simulink subsystem "INV_PWMsyncTask"  (R2022b)
settings: Solver=VariableStepAuto  StartTime=0.0  StopTime=10.0  RelTol=1e-3
values from neighbouring files (symbols this model uses):
  DPWM0Duclamp = [0 0 0 0 0 0 0 0 0 0 0 0 ... (1024 elements, 1024x1)]    [PWMLookUp.mat]    (also in prep_DPWM0_table.m = uint8(DPWM0Duclamp))
  DPWM0Dufi = [12288 12331 12374 12417 12458 12500 12541 12581 12621 12661 12700 12739 ... (1024 elements, 1024x1)]    [PWMLookUp.mat]    (also in prep_DPWM0_table.m = storedInteger(fixedPointValue))
  DPWM0Dusecfi = [-8192 -8192 -8192 -8192 -8192 -8192 -8192 -8192 -8192 -8192 -8192 -8192 ... (1024 elements, 1024x1)]    [PWMLookUp.mat]    (also in prep_DPWM0_table.m = storedInteger(fixedPointValue))
  DPWM0Dvclamp = [0 0 0 0 0 0 0 0 0 0 0 0 ... (1024 elements, 1024x1)]    [PWMLookUp.mat]    (also in prep_DPWM0_table.m = uint8(DPWM0Dvclamp))
  DPWM0Dvfi = [0 87 174 261 348 435 522 609 696 783 870 957 ... (1024 elements, 1024x1)]    [PWMLookUp.mat]    (also in prep_DPWM0_table.m = storedInteger(fixedPointValue))
  DPWM0Dvsecfi = [-8192 -8192 -8192 -8192 -8192 -8192 -8192 -8192 -8192 -8192 -8192 -8192 ... (1024 elements, 1024x1)]    [PWMLookUp.mat]    (also in prep_DPWM0_table.m = storedInteger(fixedPointValue))
  DPWM0Dwclamp = [2 2 2 2 2 2 2 2 2 2 2 2 ... (1024 elements, 1024x1)]    [PWMLookUp.mat]    (also in prep_DPWM0_table.m = uint8(DPWM0Dwclamp))
  DPWM0Dwfi = [0 0 0 0 0 0 0 0 0 0 0 0 ... (1024 elements, 1024x1)]    [PWMLookUp.mat]    (also in prep_DPWM0_table.m = storedInteger(fixedPointValue))
  DPWM0Dwsecfi = [-8192 -8192 -8192 -8192 -8192 -8192 -8192 -8192 -8192 -8192 -8192 -8192 ... (1024 elements, 1024x1)]    [PWMLookUp.mat]    (also in prep_DPWM0_table.m = storedInteger(fixedPointValue))
  DPWM1Duclamp = [1 1 1 1 1 1 1 1 1 1 1 1 ... (1024 elements, 1024x1)]    [PWMLookUp.mat]    (also in prep_DPWM1_table.m = uint8(DPWM1Duclamp))
  DPWM1Dufi = [0 0 0 0 0 0 0 0 0 0 0 0 ... (1024 elements, 1024x1)]    [PWMLookUp.mat]    (also in prep_DPWM1_table.m = storedInteger(fixedPointValue))
  DPWM1Dusecfi = [8192 8192 8192 8192 8192 8192 8192 8192 8192 8192 8192 8192 ... (1024 elements, 1024x1)]    [PWMLookUp.mat]    (also in prep_DPWM1_table.m = storedInteger(fixedPointValue))
  DPWM1Dvclamp = [0 0 0 0 0 0 0 0 0 0 0 0 ... (1024 elements, 1024x1)]    [PWMLookUp.mat]    (also in prep_DPWM1_table.m = uint8(DPWM1Dvclamp))
  DPWM1Dvfi = [-12288 -12244 -12200 -12155 -12110 -12065 -12019 -11972 -11925 -11878 -11830 -11782 ... (1024 elements, 1024x1)]    [PWMLookUp.mat]    (also in prep_DPWM1_table.m = storedInteger(fixedPointValue))
  DPWM1Dvsecfi = [8192 8192 8192 8192 8192 8192 8192 8192 8192 8192 8192 8192 ... (1024 elements, 1024x1)]    [PWMLookUp.mat]    (also in prep_DPWM1_table.m = storedInteger(fixedPointValue))
  DPWM1Dwclamp = [0 0 0 0 0 0 0 0 0 0 0 0 ... (1024 elements, 1024x1)]    [PWMLookUp.mat]    (also in prep_DPWM1_table.m = uint8(DPWM1Dwclamp))
  DPWM1Dwfi = [-12288 -12331 -12374 -12417 -12458 -12500 -12541 -12581 -12621 -12661 -12700 -12739 ... (1024 elements, 1024x1)]    [PWMLookUp.mat]    (also in prep_DPWM1_table.m = storedInteger(fixedPointValue))
  DPWM1Dwsecfi = [8192 8192 8192 8192 8192 8192 8192 8192 8192 8192 8192 8192 ... (1024 elements, 1024x1)]    [PWMLookUp.mat]    (also in prep_DPWM1_table.m = storedInteger(fixedPointValue))
  DPWM2Duclamp = [1 1 1 1 1 1 1 1 1 1 1 1 ... (1024 elements, 1024x1)]    [PWMLookUp.mat]    (also in prep_DPWM2_table.m = uint8(DPWM2Duclamp))
  DPWM2Dufi = [0 0 0 0 0 0 0 0 0 0 0 0 ... (1024 elements, 1024x1)]    [PWMLookUp.mat]    (also in prep_DPWM2_table.m = storedInteger(fixedPointValue))
  DPWM2Dusecfi = [8192 8192 8192 8192 8192 8192 8192 8192 8192 8192 8192 8192 ... (1024 elements, 1024x1)]    [PWMLookUp.mat]    (also in prep_DPWM2_table.m = storedInteger(fixedPointValue))
  DPWM2Dvclamp = [0 0 0 0 0 0 0 0 0 0 0 0 ... (1024 elements, 1024x1)]    [PWMLookUp.mat]    (also in prep_DPWM2_table.m = uint8(DPWM2Dvclamp))
  DPWM2Dvfi = [-12288 -12244 -12200 -12155 -12110 -12065 -12019 -11972 -11925 -11878 -11830 -11782 ... (1024 elements, 1024x1)]    [PWMLookUp.mat]    (also in prep_DPWM2_table.m = storedInteger(fixedPointValue))
  DPWM2Dvsecfi = [8192 8192 8192 8192 8192 8192 8192 8192 8192 8192 8192 8192 ... (1024 elements, 1024x1)]    [PWMLookUp.mat]    (also in prep_DPWM2_table.m = storedInteger(fixedPointValue))
  DPWM2Dwclamp = [0 0 0 0 0 0 0 0 0 0 0 0 ... (1024 elements, 1024x1)]    [PWMLookUp.mat]    (also in prep_DPWM2_table.m = uint8(DPWM2Dwclamp))
  DPWM2Dwfi = [-12288 -12331 -12374 -12417 -12458 -12500 -12541 -12581 -12621 -12661 -12700 -12739 ... (1024 elements, 1024x1)]    [PWMLookUp.mat]    (also in prep_DPWM2_table.m = storedInteger(fixedPointValue))
  DPWM2Dwsecfi = [8192 8192 8192 8192 8192 8192 8192 8192 8192 8192 8192 8192 ... (1024 elements, 1024x1)]    [PWMLookUp.mat]    (also in prep_DPWM2_table.m = storedInteger(fixedPointValue))
  DPWM3Duclamp = [0 0 0 0 0 0 0 0 0 0 0 0 ... (1024 elements, 1024x1)]    [PWMLookUp.mat]    (also in prep_DPWM3_table.m = uint8(DPWM3Duclamp))
  DPWM3Dufi = [12288 12331 12374 12417 12458 12500 12541 12581 12621 12661 12700 12739 ... (1024 elements, 1024x1)]    [PWMLookUp.mat]    (also in prep_DPWM3_table.m = storedInteger(fixedPointValue))
  DPWM3Dusecfi = [-8192 -8192 -8192 -8192 -8192 -8192 -8192 -8192 -8192 -8192 -8192 -8192 ... (1024 elements, 1024x1)]    [PWMLookUp.mat]    (also in prep_DPWM3_table.m = storedInteger(fixedPointValue))
  DPWM3Dvclamp = [0 0 0 0 0 0 0 0 0 0 0 0 ... (1024 elements, 1024x1)]    [PWMLookUp.mat]    (also in prep_DPWM3_table.m = uint8(DPWM3Dvclamp))
  DPWM3Dvfi = [0 87 174 261 348 435 522 609 696 783 870 957 ... (1024 elements, 1024x1)]    [PWMLookUp.mat]    (also in prep_DPWM3_table.m = storedInteger(fixedPointValue))
  DPWM3Dvsecfi = [-8192 -8192 -8192 -8192 -8192 -8192 -8192 -8192 -8192 -8192 -8192 -8192 ... (1024 elements, 1024x1)]    [PWMLookUp.mat]    (also in prep_DPWM3_table.m = storedInteger(fixedPointValue))
  DPWM3Dwclamp = [2 2 2 2 2 2 2 2 2 2 2 2 ... (1024 elements, 1024x1)]    [PWMLookUp.mat]    (also in prep_DPWM3_table.m = uint8(DPWM3Dwclamp))
  DPWM3Dwfi = [0 0 0 0 0 0 0 0 0 0 0 0 ... (1024 elements, 1024x1)]    [PWMLookUp.mat]    (also in prep_DPWM3_table.m = storedInteger(fixedPointValue))
  DPWM3Dwsecfi = [-8192 -8192 -8192 -8192 -8192 -8192 -8192 -8192 -8192 -8192 -8192 -8192 ... (1024 elements, 1024x1)]    [PWMLookUp.mat]    (also in prep_DPWM3_table.m = storedInteger(fixedPointValue))
  DPWMmaxDuclamp = [1 1 1 1 1 1 1 1 1 1 1 1 ... (1024 elements, 1024x1)]    [PWMLookUp.mat]    (also in prep_DPWMmax_table.m = uint8(DPWMmaxDuclamp))
  DPWMmaxDufi = [0 0 0 0 0 0 0 0 0 0 0 0 ... (1024 elements, 1024x1)]    [PWMLookUp.mat]    (also in prep_DPWMmax_table.m = storedInteger(fixedPointValue))
  DPWMmaxDusecfi = [8192 8192 8192 8192 8192 8192 8192 8192 8192 8192 8192 8192 ... (1024 elements, 1024x1)]    [PWMLookUp.mat]    (also in prep_DPWMmax_table.m = storedInteger(fixedPointValue))
  DPWMmaxDvclamp = [0 0 0 0 0 0 0 0 0 0 0 0 ... (1024 elements, 1024x1)]    [PWMLookUp.mat]    (also in prep_DPWMmax_table.m = uint8(DPWMmaxDvclamp))
  DPWMmaxDvfi = [-12288 -12244 -12200 -12155 -12110 -12065 -12019 -11972 -11925 -11878 -11830 -11782 ... (1024 elements, 1024x1)]    [PWMLookUp.mat]    (also in prep_DPWMmax_table.m = storedInteger(fixedPointValue))
  DPWMmaxDvsecfi = [8192 8192 8192 8192 8192 8192 8192 8192 8192 8192 8192 8192 ... (1024 elements, 1024x1)]    [PWMLookUp.mat]    (also in prep_DPWMmax_table.m = storedInteger(fixedPointValue))
  DPWMmaxDwclamp = [0 0 0 0 0 0 0 0 0 0 0 0 ... (1024 elements, 1024x1)]    [PWMLookUp.mat]    (also in prep_DPWMmax_table.m = uint8(DPWMmaxDwclamp))
  DPWMmaxDwfi = [-12288 -12331 -12374 -12417 -12458 -12500 -12541 -12581 -12621 -12661 -12700 -12739 ... (1024 elements, 1024x1)]    [PWMLookUp.mat]    (also in prep_DPWMmax_table.m = storedInteger(fixedPointValue))
  DPWMmaxDwsecfi = [8192 8192 8192 8192 8192 8192 8192 8192 8192 8192 8192 8192 ... (1024 elements, 1024x1)]    [PWMLookUp.mat]    (also in prep_DPWMmax_table.m = storedInteger(fixedPointValue))
  DPWMminDuclamp = [0 0 0 0 0 0 0 0 0 0 0 0 ... (1024 elements, 1024x1)]    [PWMLookUp.mat]    (also in prep_DPWMmin_table.m = uint8(DPWMminDuclamp))
  DPWMminDufi = [12288 12331 12374 12417 12458 12500 12541 12581 12621 12661 12700 12739 ... (1024 elements, 1024x1)]    [PWMLookUp.mat]    (also in prep_DPWMmin_table.m = storedInteger(fixedPointValue))
  DPWMminDusecfi = [-8192 -8192 -8192 -8192 -8192 -8192 -8192 -8192 -8192 -8192 -8192 -8192 ... (1024 elements, 1024x1)]    [PWMLookUp.mat]    (also in prep_DPWMmin_table.m = storedInteger(fixedPointValue))
  DPWMminDvclamp = [0 0 0 0 0 0 0 0 0 0 0 0 ... (1024 elements, 1024x1)]    [PWMLookUp.mat]    (also in prep_DPWMmin_table.m = uint8(DPWMminDvclamp))
  DPWMminDvfi = [0 87 174 261 348 435 522 609 696 783 870 957 ... (1024 elements, 1024x1)]    [PWMLookUp.mat]    (also in prep_DPWMmin_table.m = storedInteger(fixedPointValue))
  DPWMminDvsecfi = [-8192 -8192 -8192 -8192 -8192 -8192 -8192 -8192 -8192 -8192 -8192 -8192 ... (1024 elements, 1024x1)]    [PWMLookUp.mat]    (also in prep_DPWMmin_table.m = storedInteger(fixedPointValue))
  DPWMminDwclamp = [2 2 2 2 2 2 2 2 2 2 2 2 ... (1024 elements, 1024x1)]    [PWMLookUp.mat]    (also in prep_DPWMmin_table.m = uint8(DPWMminDwclamp))
  DPWMminDwfi = [0 0 0 0 0 0 0 0 0 0 0 0 ... (1024 elements, 1024x1)]    [PWMLookUp.mat]    (also in prep_DPWMmin_table.m = storedInteger(fixedPointValue))
  DPWMminDwsecfi = [-8192 -8192 -8192 -8192 -8192 -8192 -8192 -8192 -8192 -8192 -8192 -8192 ... (1024 elements, 1024x1)]    [PWMLookUp.mat]    (also in prep_DPWMmin_table.m = storedInteger(fixedPointValue))
  SPWMDufi = [8192 8192 8191 8191 8190 8188 8186 8184 8182 8180 8177 8173 ... (1024 elements, 1024x1)]    [PWMLookUp.mat]    (also in prep_SinePWM_table.m = storedInteger(fixedPointValue))
  SPWMDvfi = [-4096 -4052 -4009 -3965 -3921 -3876 -3832 -3788 -3743 -3698 -3653 -3608 ... (1024 elements, 1024x1)]    [PWMLookUp.mat]    (also in prep_SinePWM_table.m = storedInteger(fixedPointValue))
  SPWMDwfi = [-4096 -4139 -4183 -4226 -4269 -4312 -4354 -4397 -4439 -4481 -4523 -4565 ... (1024 elements, 1024x1)]    [PWMLookUp.mat]    (also in prep_SinePWM_table.m = storedInteger(fixedPointValue))
  SVPWMDufi = [6144 6166 6187 6208 6229 6250 6270 6291 6311 6330 6350 6369 ... (1024 elements, 1024x1)]    [PWMLookUp.mat]    (also in prep_SVPWM_table.m = storedInteger(fixedPointValue))
  SVPWMDvfi = [-6144 -6079 -6013 -5947 -5881 -5815 -5748 -5681 -5614 -5547 -5480 -5412 ... (1024 elements, 1024x1)]    [PWMLookUp.mat]    (also in prep_SVPWM_table.m = storedInteger(fixedPointValue))
  SVPWMDwfi = [-6144 -6166 -6187 -6208 -6229 -6250 -6270 -6291 -6311 -6330 -6350 -6369 ... (1024 elements, 1024x1)]    [PWMLookUp.mat]    (also in prep_SVPWM_table.m = storedInteger(fixedPointValue))
  THISPWMDufi = [6823 6823 6823 6823 6824 6825 6826 6827 6828 6829 6831 6832 ... (1024 elements, 1024x1)]    [PWMLookUp.mat]    (also in prep_THISPWM_table.m = storedInteger(fixedPointValue))
  THISPWMDvfi = [-5465 -5421 -5377 -5332 -5286 -5240 -5193 -5145 -5097 -5049 -4999 -4949 ... (1024 elements, 1024x1)]    [PWMLookUp.mat]    (also in prep_THISPWM_table.m = storedInteger(fixedPointValue))
  THISPWMDwfi = [-5465 -5508 -5551 -5593 -5634 -5675 -5715 -5755 -5794 -5832 -5869 -5906 ... (1024 elements, 1024x1)]    [PWMLookUp.mat]    (also in prep_THISPWM_table.m = storedInteger(fixedPointValue))
libraries: simulink x16
(part 1 of 2)
settings Model: Creator=ReiterTo  LastModifiedBy=ReiterTo

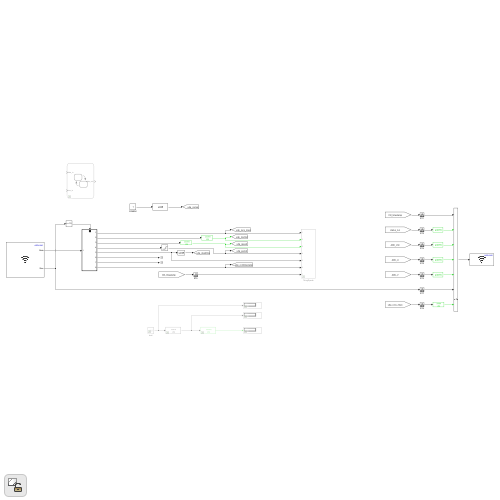
[thumbnail: Simulink's stored preview of the top-level diagram]
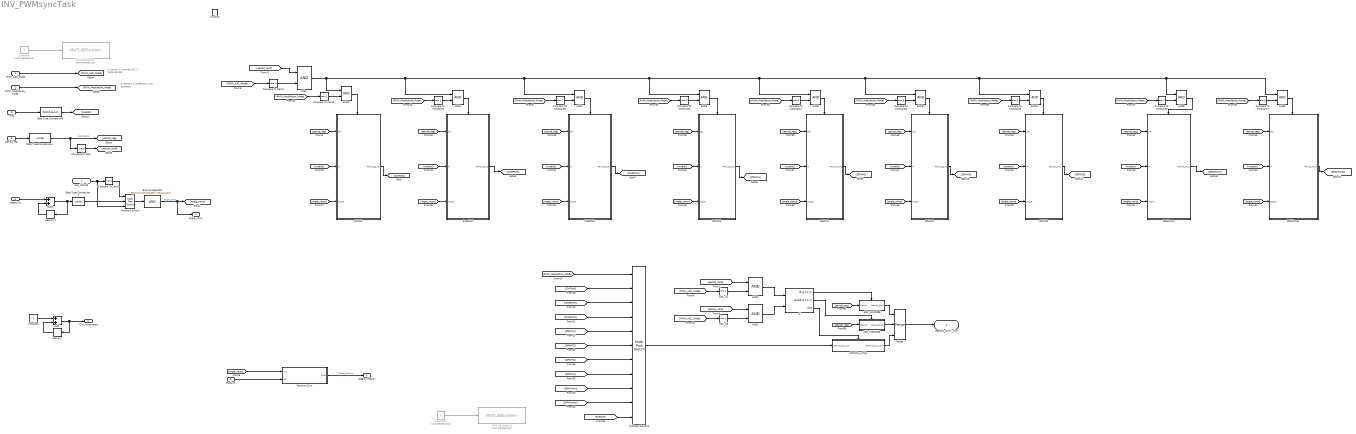
== system INV_PWMsyncTask ==
  note: 0: SVPWM
      | 1: SinePWM
      | 2: not available
  note: 0: normal
      | 1: lowside ASC
      | 2: highside ASC
  PWM_ASC_Mode : Inport  OutDataTypeStr=uint8  PortDimensions=1
  PWM_Modulation_Mode : Inport  Port=2  OutDataTypeStr=uint8  PortDimensions=1
  mod : Inport  Port=3  OutDataTypeStr=fixdt(0,16,14)  PortDimensions=1
  speed_inc : Inport  Port=4  OutDataTypeStr=fixdt(0,32,16)  PortDimensions=1
  period_reg : Inport  Port=5  OutDataTypeStr=uint16  PortDimensions=1
  PosSync : Inport  Port=6  OutDataTypeStr=uint16  PortDimensions=1
  pos_hillhold : Inport  Port=7  OutDataTypeStr=uint16  PortDimensions=1
  function : TriggerPort  TriggerType=function-call  VariantControl=(inherit)  PortDimensions=1
  AND{,1..11} (12 alike) : Logic  AllPortsSameDT=off  OutDataTypeStr=boolean
  ASC_HIGHSIDE : Subsystem  TreatAsAtomicUnit=on
  ASC_HS : simulink/Logic and Bit Operations/Compare To Constant  relop===  const=2  OutDataTypeStr=boolean
  ASC_LOWSIDE : Subsystem  TreatAsAtomicUnit=on
  ASC_LS : simulink/Logic and Bit Operations/Compare To Constant  relop===  const=1  OutDataTypeStr=boolean
  Add : Sum
  Add1 : Sum
  Bitwise Operator : simulink/Logic and Bit Operations/Bitwise Operator  logicop=AND  UseBitMask=on  BitMask=bin2dec('1111111111')  BitMaskRealWorld=Stored Integer
  Compare To Constant2 : simulink/Logic and Bit Operations/Compare To Constant  relop===  const=1  OutDataTypeStr=boolean
  Compare To Constant3 : simulink/Logic and Bit Operations/Compare To Constant  relop===  const=3  OutDataTypeStr=boolean
  Compare To Constant4 : simulink/Logic and Bit Operations/Compare To Constant  relop===  const=4  OutDataTypeStr=boolean
  Compare To Constant5 : simulink/Logic and Bit Operations/Compare To Constant  relop===  const=2  OutDataTypeStr=boolean
  Compare To Constant6 : simulink/Logic and Bit Operations/Compare To Constant  relop===  const=7  OutDataTypeStr=boolean
  Compare To Constant7 : simulink/Logic and Bit Operations/Compare To Constant  relop===  const=8  OutDataTypeStr=boolean
  Compare To Constant8 : simulink/Logic and Bit Operations/Compare To Constant  relop===  const=5  OutDataTypeStr=boolean
  Compare To Constant9 : simulink/Logic and Bit Operations/Compare To Constant  relop===  const=6  OutDataTypeStr=boolean
  Compare To Zero : simulink/Logic and Bit Operations/Compare To Zero  relop=~=  OutDataTypeStr=boolean
  Compare To Zero1 : simulink/Logic and Bit Operations/Compare To Zero  relop===  OutDataTypeStr=boolean
  Compare To Zero2 : simulink/Logic and Bit Operations/Compare To Zero  relop=~=  OutDataTypeStr=uint8
  Compare To Zero3 : simulink/Logic and Bit Operations/Compare To Zero  relop===  OutDataTypeStr=boolean
  Constant : Constant  OutDataTypeStr=uint32  SampleTime=-1
  Constant1 : Constant  Priority=1  Commented=on  OutDataTypeStr=uint8  SampleTime=-1
  Constant2 : Constant  Commented=on  Value=0  OutDataTypeStr=uint8  SampleTime=-1
  DPWM0 : Subsystem
      settings: RTWSystemCode=Inline
  DPWM1 : Subsystem
      settings: RTWSystemCode=Inline
  DPWM2 : Subsystem
      settings: RTWSystemCode=Inline
  DPWM3 : Subsystem
      settings: RTWSystemCode=Inline
  DPWMmax : Subsystem
      settings: RTWSystemCode=Inline
  DPWMmin : Subsystem
      settings: RTWSystemCode=Inline
  Data Type Conversion1 : DataTypeConversion  OutDataTypeStr=uint16  RndMeth=Simplest  SaturateOnIntegerOverflow=off
  Data Type Conversion4 : DataTypeConversion  OutDataTypeStr=uint16  RndMeth=Simplest  SaturateOnIntegerOverflow=off
  Data Type Conversion6 : DataTypeConversion  OutDataTypeStr=fixdt(0,16,14)  SaturateOnIntegerOverflow=off  RndMeth=Floor
  If : If  NumInputs=2  IfExpression=u1 == 1  ElseIfExpressions=u2 == 1
  MATLAB System : MATLABSystem  Commented=on  System=invIOfastRX1
      mask Type: invIOfastRX1
      mask Display:
      | disp('Arduino Nano 33 IoT \n IO 1 RX FAST');
      | port_label('input',1,'pegel');
  MATLAB System1 : MATLABSystem  Commented=on  System=invIOfastRX1
      mask Type: invIOfastRX1
      mask Display:
      | disp('Arduino Nano 33 IoT \n IO 1 RX FAST');
      | port_label('input',1,'pegel');
  Memory : Memory  InheritSampleTime=on  LinearizeMemory=on  StateName=ctrl_timestamp_z1
  Memory1 : Memory  InheritSampleTime=on  LinearizeMemory=on  StateName=ctrl_timestamp_z1
  Merge : Merge  Inputs=3
  Multiport Switch : MultiPortSwitch  DataPortOrder=Zero-based contiguous  Inputs=2  zeroidx=on  SaturateOnIntegerOverflow=off  InputSameDT=off
  Multiport Switch1 : MultiPortSwitch  DataPortOrder=Zero-based contiguous  Inputs=9  DataPortForDefault=Additional data port  zeroidx=on  RndMeth=Simplest  SaturateOnIntegerOverflow=off  InputSameDT=off
  NORMAL_PWM : Subsystem  TreatAsAtomicUnit=on
  Position_Sync : Subsystem
  SVPWM : Subsystem
      settings: RTWSystemCode=Inline
  SinePWM : Subsystem
      settings: RTWSystemCode=Inline
  THISPWM : Subsystem
      settings: RTWSystemCode=Inline
  Ctrl_timestamp : Outport  OutDataTypeStr=uint32  PortDimensions=1
  PERIOD_DUTY_OUT : Outport  Port=2  OutDataTypeStr=uint16  InitialOutput=[uint16(5000),uint16(2500),uint16(2500),uint16(2500)]
  toggle_rotation : Outport  Port=3  OutDataTypeStr=uint16  PortDimensions=1
  angle_ramp : Outport  Port=4  OutDataTypeStr=uint16  PortDimensions=1
  wires:
  Compare To Constant4/1 -> AND6/2
  [PWM_Modulation_Mode] -> Compare To Zero3/1
  AND6/1 -> DPWM2/Enable
  AND1/1 -> If/1
  Compare To Zero/1 -> [period_valid]
  Compare To Zero2/1 -> Multiport Switch/1
  [angle_ramp] -> Position_Sync/1(In1)
  [PWM_Modulation_Mode] -> Compare To Constant3/1
  [period_valid] -> AND/1
  [PWM_Modulation_Mode] -> Compare To Constant4/1
  [PWM_ASC_Mode] -> ASC_LS/1
  Compare To Constant3/1 -> AND5/2
  AND3/1 -> SVPWM/Enable
  mod/1 -> Data Type Conversion6/1
  pos_hillhold/1 -> Compare To Zero2/1, Multiport Switch/3
  Compare To Constant2/1 -> AND4/2
  Memory/1 -> Add/2
  [PWM_Modulation_Mode] -> Compare To Constant2/1
  Add/1 -> Memory/1, Ctrl_timestamp/1
  Memory1/1 -> Add1/2
  ASC_LS/1 -> AND1/2
  period_reg/1 -> Data Type Conversion4/1
  PWM_ASC_Mode/1 -> [PWM_ASC_Mode]
  Constant2/1 -> MATLAB System1/1
  Multiport Switch/1 -> Bitwise Operator/1
  [PWM_ASC_Mode] -> ASC_HS/1
  PosSync/1 -> Position_Sync/2(In2)
  [PWM_ASC_Mode] -> Compare To Zero1/1
  Add1/1 -> Data Type Conversion1/1, Memory1/1
  [period_valid] -> AND2/1
  Compare To Zero3/1 -> AND3/2
  AND5/1 -> DPWM1/Enable
  ASC_HS/1 -> AND2/2
  PWM_Modulation_Mode/1 -> [PWM_Modulation_Mode]
  Compare To Zero1/1 -> AND/2
  Constant/1 -> Add/1
  [period_valid] -> AND1/1
  Bitwise Operator/1 -> [angle_ramp], angle_ramp/1  "angle_ramp"
  speed_inc/1 -> Add1/1
  AND2/1 -> If/2
  Position_Sync/1(Out1) -> toggle_rotation/1  "Phase_polarity"
  Data Type Conversion4/1 -> Compare To Zero/1, [period_reg]  "period_sig"
  [period_reg] -> SVPWM/1(per)
  Constant1/1 -> MATLAB System/1
  [modidx] -> SVPWM/2(M)
  Data Type Conversion1/1 -> Multiport Switch/2
  AND4/1 -> SinePWM/Enable
  AND7/1 -> THISPWM/Enable
  Compare To Constant5/1 -> AND7/2
  [PWM_Modulation_Mode] -> Compare To Constant5/1
  Multiport Switch1/1 -> NORMAL_PWM/1(Period_Duty_IN)
  [PWM_Modulation_Mode] -> Multiport Switch1/1
  Compare To Constant6/1 -> AND8/2
  AND8/1 -> DPWMmin/Enable
  [PWM_Modulation_Mode] -> Compare To Constant6/1
  AND9/1 -> DPWMmax/Enable
  Compare To Constant7/1 -> AND9/2
  [PWM_Modulation_Mode] -> Compare To Constant7/1
  [SVPWM] -> Multiport Switch1/2
  [SinePWM] -> Multiport Switch1/3
  [THISPWM] -> Multiport Switch1/4
  [DPWM1] -> Multiport Switch1/5
  [DPWM2] -> Multiport Switch1/6
  Data Type Conversion6/1 -> [modidx]
  [angle_ramp] -> SVPWM/3(angle)
  [period_reg] -> SinePWM/1(per)
  [angle_ramp] -> SinePWM/3(angle)
  [modidx] -> SinePWM/2(M)
  [modidx] -> THISPWM/2(M)
  [angle_ramp] -> THISPWM/3(angle)
  [period_reg] -> THISPWM/1(per)
  [angle_ramp] -> DPWM1/3(angle)
  [period_reg] -> DPWM1/1(per)
  [modidx] -> DPWM1/2(M)
  [angle_ramp] -> DPWM2/3(angle)
  [period_reg] -> DPWM2/1(per)
  [modidx] -> DPWM2/2(M)
  [angle_ramp] -> DPWMmin/3(angle)
  [period_reg] -> DPWMmin/1(per)
  [modidx] -> DPWMmin/2(M)
  [angle_ramp] -> DPWMmax/3(angle)
  [period_reg] -> DPWMmax/1(per)
  [modidx] -> DPWMmax/2(M)
  [modidx] -> DPWM0/2(M)
  [period_reg] -> DPWM0/1(per)
  AND10/1 -> DPWM0/Enable
  [PWM_Modulation_Mode] -> Compare To Constant8/1
  Compare To Constant8/1 -> AND10/2
  [angle_ramp] -> DPWM0/3(angle)
  [modidx] -> DPWM3/2(M)
  [period_reg] -> DPWM3/1(per)
  AND/1 -> AND6/1, AND8/1, AND9/1, AND11/1, AND10/1, AND5/1, AND7/1, AND4/1, AND3/1
  AND11/1 -> DPWM3/Enable
  [PWM_Modulation_Mode] -> Compare To Constant9/1
  Compare To Constant9/1 -> AND11/2
  [angle_ramp] -> DPWM3/3(angle)
  [DPWMmax] -> Multiport Switch1/10
  [DPWMmin] -> Multiport Switch1/9
  [DPWM0] -> Multiport Switch1/7
  [DPWM3] -> Multiport Switch1/8
  [SVPWM] -> Multiport Switch1/11
  If/1 -> ASC_LOWSIDE/Action
  If/2 -> ASC_HIGHSIDE/Action
  If/3 -> NORMAL_PWM/Action
  ASC_LOWSIDE/1(Period_Duty) -> Merge/1
  [period_reg] -> ASC_LOWSIDE/1(Period)
  [period_reg] -> ASC_HIGHSIDE/1(Period)
  ASC_HIGHSIDE/1(Period_Duty) -> Merge/2
  NORMAL_PWM/1(Period_Duty_OUT) -> Merge/3
  Merge/1 -> PERIOD_DUTY_OUT/1
  SVPWM/1(Period_Duty) -> [SVPWM]
  SinePWM/1(Period_Duty) -> [SinePWM]
  DPWM1/1(Period_Duty) -> [DPWM1]
  DPWM2/1(Period_Duty) -> [DPWM2]
  DPWM0/1(Period_Duty) -> [DPWM0]
  DPWM3/1(Period_Duty) -> [DPWM3]
  DPWMmin/1(Period_Duty) -> [DPWMmin]
  DPWMmax/1(Period_Duty) -> [DPWMmax]
  THISPWM/1(Period_Duty) -> [THISPWM]

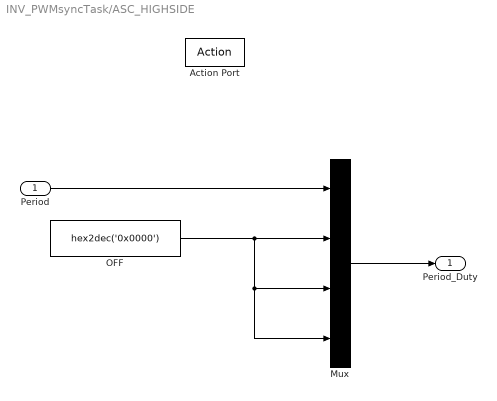
== system INV_PWMsyncTask/ASC_HIGHSIDE ==
  Period : Inport
  Action Port : ActionPort
  Mux : Mux
  OFF : Constant  Value=hex2dec('0x0000')  OutDataTypeStr=uint16  SampleTime=-1
  Period_Duty : Outport
  wires:
  Period/1 -> Mux/1
  Mux/1 -> Period_Duty/1
  OFF/1 -> Mux/3, Mux/4, Mux/2

== system INV_PWMsyncTask/ASC_LOWSIDE ==
  Period : Inport
  Action Port : ActionPort
  Mux : Mux
  ON : Constant  Value=hex2dec('0xFFFF')  OutDataTypeStr=uint16  SampleTime=-1
  Period_Duty : Outport
  wires:
  Mux/1 -> Period_Duty/1
  ON/1 -> Mux/3, Mux/4, Mux/2
  Period/1 -> Mux/1

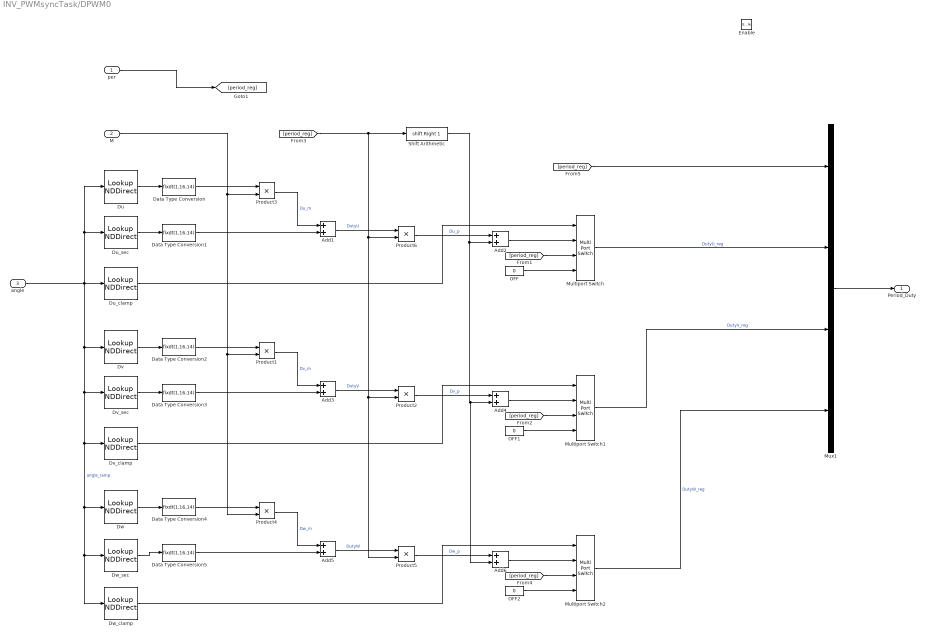
== system INV_PWMsyncTask/DPWM0 ==
  per : Inport
  M : Inport  Port=2
  angle : Inport  Port=3
  Enable : EnablePort
  Add1 : Sum  RndMeth=Simplest  OutDataTypeStr=Inherit: Same as first input
  Add2 : Sum  OutDataTypeStr=uint16  RndMeth=Simplest  SaturateOnIntegerOverflow=on
  Add3 : Sum  RndMeth=Simplest  OutDataTypeStr=Inherit: Same as first input
  Add4 : Sum  OutDataTypeStr=uint16  RndMeth=Simplest  SaturateOnIntegerOverflow=on
  Add5 : Sum  RndMeth=Simplest  OutDataTypeStr=Inherit: Same as first input
  Add6 : Sum  OutDataTypeStr=uint16  RndMeth=Simplest  SaturateOnIntegerOverflow=on
  Data Type Conversion{,1..5} (6 alike) : DataTypeConversion  OutDataTypeStr=fixdt(1,16,14)  ConvertRealWorld=Stored Integer (SI)  RndMeth=Simplest  SaturateOnIntegerOverflow=off
  Du : LookupNDDirect  NumberOfTableDimensions=1  Table=DPWM0Dufi  DiagnosticForOutOfRangeInput=None  RemoveProtectionInput=on  TableDataTypeStr=int16
      settings: LockScale=on
  Du_clamp : LookupNDDirect  NumberOfTableDimensions=1  Table=DPWM0Duclamp  RemoveProtectionInput=on  TableDataTypeStr=uint8
      settings: LockScale=on
  Du_sec : LookupNDDirect  NumberOfTableDimensions=1  Table=DPWM0Dusecfi  RemoveProtectionInput=on  TableDataTypeStr=int16
      settings: LockScale=on
  Dv : LookupNDDirect  NumberOfTableDimensions=1  Table=DPWM0Dvfi  DiagnosticForOutOfRangeInput=None  RemoveProtectionInput=on  TableDataTypeStr=int16
      settings: LockScale=on
  Dv_clamp : LookupNDDirect  NumberOfTableDimensions=1  Table=DPWM0Dvclamp  RemoveProtectionInput=on  TableDataTypeStr=uint8
      settings: LockScale=on
  Dv_sec : LookupNDDirect  NumberOfTableDimensions=1  Table=DPWM0Dvsecfi  RemoveProtectionInput=on  TableDataTypeStr=int16
      settings: LockScale=on
  Dw : LookupNDDirect  NumberOfTableDimensions=1  Table=DPWM0Dwfi  DiagnosticForOutOfRangeInput=None  RemoveProtectionInput=on  TableDataTypeStr=int16
      settings: LockScale=on
  Dw_clamp : LookupNDDirect  NumberOfTableDimensions=1  Table=DPWM0Dwclamp  RemoveProtectionInput=on  TableDataTypeStr=uint8
      settings: LockScale=on
  Dw_sec : LookupNDDirect  NumberOfTableDimensions=1  Table=DPWM0Dwsecfi  RemoveProtectionInput=on  TableDataTypeStr=int16
      settings: LockScale=on
  Multiport Switch : MultiPortSwitch  DataPortOrder=Zero-based contiguous  DiagnosticForDefault=None  zeroidx=on  SaturateOnIntegerOverflow=off  InputSameDT=off
  Multiport Switch1 : MultiPortSwitch  DataPortOrder=Zero-based contiguous  DiagnosticForDefault=None  zeroidx=on  SaturateOnIntegerOverflow=off  InputSameDT=off
  Multiport Switch2 : MultiPortSwitch  DataPortOrder=Zero-based contiguous  DiagnosticForDefault=None  zeroidx=on  SaturateOnIntegerOverflow=off  InputSameDT=off
  Mux1 : Mux
  OFF : Constant  Value=0  OutDataTypeStr=uint16  SampleTime=-1
  OFF1 : Constant  Value=0  OutDataTypeStr=uint16  SampleTime=-1
  OFF2 : Constant  Value=0  OutDataTypeStr=uint16  SampleTime=-1
  Product1 : Product  RndMeth=Simplest  OutDataTypeStr=Inherit: Same as first input  LockScale=on
  Product2 : Product  OutDataTypeStr=int16  RndMeth=Simplest
  Product3 : Product  RndMeth=Simplest  OutDataTypeStr=Inherit: Same as first input  LockScale=on
  Product4 : Product  RndMeth=Simplest  OutDataTypeStr=Inherit: Same as first input  LockScale=on
  Product5 : Product  OutDataTypeStr=int16  RndMeth=Simplest
  Product6 : Product  OutDataTypeStr=int16  RndMeth=Simplest
  Shift Arithmetic : ArithShift  BitShiftNumber=1  BitShiftDirection=Right
  Period_Duty : Outport
  wires:
  [period_reg] -> Mux1/1
  Multiport Switch/1 -> Mux1/2  "DutyU_reg"
  Multiport Switch1/1 -> Mux1/3  "DutyV_reg"
  Multiport Switch2/1 -> Mux1/4  "DutyW_reg"
  Mux1/1 -> Period_Duty/1
  per/1 -> [period_reg]
  Add2/1 -> Multiport Switch/2
  Data Type Conversion/1 -> Product3/1
  Product6/1 -> Add2/1  "Du_p"
  Du/1 -> Data Type Conversion/1
  Product3/1 -> Add1/1  "Du_m"
  Du_sec/1 -> Data Type Conversion1/1
  Add1/1 -> Product6/1  "DutyU"
  [period_reg] -> Multiport Switch/3
  OFF/1 -> Multiport Switch/4
  Du_clamp/1 -> Multiport Switch/1
  Data Type Conversion1/1 -> Add1/2
  Dv_clamp/1 -> Multiport Switch1/1
  Product1/1 -> Add3/1  "Dv_m"
  OFF1/1 -> Multiport Switch1/4
  Data Type Conversion3/1 -> Add3/2
  Add4/1 -> Multiport Switch1/2
  Data Type Conversion2/1 -> Product1/1
  Add3/1 -> Product2/1  "DutyV"
  [period_reg] -> Multiport Switch1/3
  Dv/1 -> Data Type Conversion2/1
  Dv_sec/1 -> Data Type Conversion3/1
  Product2/1 -> Add4/1  "Dv_p"
  [period_reg] -> Shift Arithmetic/1, Product5/2, Product2/2, Product6/2
  Dw_sec/1 -> Data Type Conversion5/1
  M/1 -> Product4/2, Product1/2, Product3/2
  Shift Arithmetic/1 -> Add2/2, Add6/2, Add4/2
  angle/1 -> Dv_clamp/1, Dw_clamp/1, Dw_sec/1, Dw/1, Dv_sec/1, Dv/1, Du_sec/1, Du/1, Du_clamp/1  "angle_ramp"
  [period_reg] -> Multiport Switch2/3
  Data Type Conversion5/1 -> Add5/2
  Add6/1 -> Multiport Switch2/2
  Add5/1 -> Product5/1  "DutyW"
  Dw/1 -> Data Type Conversion4/1
  Dw_clamp/1 -> Multiport Switch2/1
  OFF2/1 -> Multiport Switch2/4
  Product4/1 -> Add5/1  "Dw_m"
  Data Type Conversion4/1 -> Product4/1
  Product5/1 -> Add6/1  "Dw_p"

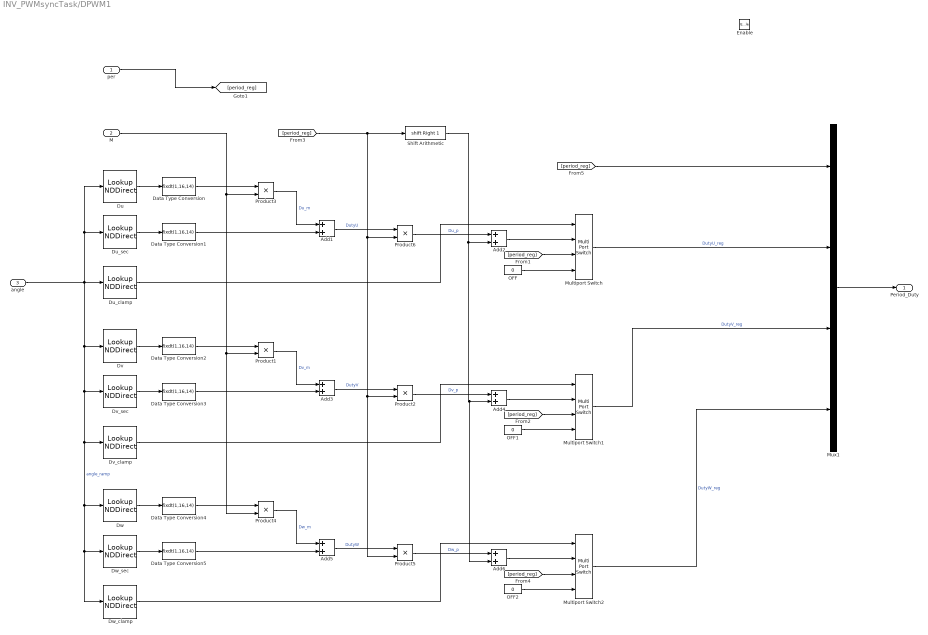
== system INV_PWMsyncTask/DPWM1 ==
  per : Inport
  M : Inport  Port=2
  angle : Inport  Port=3
  Enable : EnablePort
  Add1 : Sum  RndMeth=Simplest  OutDataTypeStr=Inherit: Same as first input
  Add2 : Sum  OutDataTypeStr=uint16  RndMeth=Simplest  SaturateOnIntegerOverflow=on
  Add3 : Sum  RndMeth=Simplest  OutDataTypeStr=Inherit: Same as first input
  Add4 : Sum  OutDataTypeStr=uint16  RndMeth=Simplest  SaturateOnIntegerOverflow=on
  Add5 : Sum  RndMeth=Simplest  OutDataTypeStr=Inherit: Same as first input
  Add6 : Sum  OutDataTypeStr=uint16  RndMeth=Simplest  SaturateOnIntegerOverflow=on
  Data Type Conversion{,1..5} (6 alike) : DataTypeConversion  OutDataTypeStr=fixdt(1,16,14)  ConvertRealWorld=Stored Integer (SI)  RndMeth=Simplest  SaturateOnIntegerOverflow=off
  Du : LookupNDDirect  NumberOfTableDimensions=1  Table=DPWM1Dufi  DiagnosticForOutOfRangeInput=None  RemoveProtectionInput=on  TableDataTypeStr=int16
      settings: LockScale=on
  Du_clamp : LookupNDDirect  NumberOfTableDimensions=1  Table=DPWM1Duclamp  RemoveProtectionInput=on  TableDataTypeStr=uint8
      settings: LockScale=on
  Du_sec : LookupNDDirect  NumberOfTableDimensions=1  Table=DPWM1Dusecfi  RemoveProtectionInput=on  TableDataTypeStr=int16
      settings: LockScale=on
  Dv : LookupNDDirect  NumberOfTableDimensions=1  Table=DPWM1Dvfi  DiagnosticForOutOfRangeInput=None  RemoveProtectionInput=on  TableDataTypeStr=int16
      settings: LockScale=on
  Dv_clamp : LookupNDDirect  NumberOfTableDimensions=1  Table=DPWM1Dvclamp  RemoveProtectionInput=on  TableDataTypeStr=uint8
      settings: LockScale=on
  Dv_sec : LookupNDDirect  NumberOfTableDimensions=1  Table=DPWM1Dvsecfi  RemoveProtectionInput=on  TableDataTypeStr=int16
      settings: LockScale=on
  Dw : LookupNDDirect  NumberOfTableDimensions=1  Table=DPWM1Dwfi  DiagnosticForOutOfRangeInput=None  RemoveProtectionInput=on  TableDataTypeStr=int16
      settings: LockScale=on
  Dw_clamp : LookupNDDirect  NumberOfTableDimensions=1  Table=DPWM1Dwclamp  RemoveProtectionInput=on  TableDataTypeStr=uint8
      settings: LockScale=on
  Dw_sec : LookupNDDirect  NumberOfTableDimensions=1  Table=DPWM1Dwsecfi  RemoveProtectionInput=on  TableDataTypeStr=int16
      settings: LockScale=on
  Multiport Switch : MultiPortSwitch  DataPortOrder=Zero-based contiguous  DiagnosticForDefault=None  zeroidx=on  SaturateOnIntegerOverflow=off  InputSameDT=off
  Multiport Switch1 : MultiPortSwitch  DataPortOrder=Zero-based contiguous  DiagnosticForDefault=None  zeroidx=on  SaturateOnIntegerOverflow=off  InputSameDT=off
  Multiport Switch2 : MultiPortSwitch  DataPortOrder=Zero-based contiguous  DiagnosticForDefault=None  zeroidx=on  SaturateOnIntegerOverflow=off  InputSameDT=off
  Mux1 : Mux
  OFF : Constant  Value=0  OutDataTypeStr=uint16  SampleTime=-1
  OFF1 : Constant  Value=0  OutDataTypeStr=uint16  SampleTime=-1
  OFF2 : Constant  Value=0  OutDataTypeStr=uint16  SampleTime=-1
  Product1 : Product  RndMeth=Simplest  OutDataTypeStr=Inherit: Same as first input  LockScale=on
  Product2 : Product  OutDataTypeStr=int16  RndMeth=Simplest
  Product3 : Product  RndMeth=Simplest  OutDataTypeStr=Inherit: Same as first input  LockScale=on
  Product4 : Product  RndMeth=Simplest  OutDataTypeStr=Inherit: Same as first input  LockScale=on
  Product5 : Product  OutDataTypeStr=int16  RndMeth=Simplest
  Product6 : Product  OutDataTypeStr=int16  RndMeth=Simplest
  Shift Arithmetic : ArithShift  BitShiftNumber=1  BitShiftDirection=Right
  Period_Duty : Outport
  wires:
  Multiport Switch2/1 -> Mux1/4  "DutyW_reg"
  [period_reg] -> Mux1/1
  Mux1/1 -> Period_Duty/1
  Multiport Switch1/1 -> Mux1/3  "DutyV_reg"
  Multiport Switch/1 -> Mux1/2  "DutyU_reg"
  per/1 -> [period_reg]
  Add2/1 -> Multiport Switch/2
  Data Type Conversion/1 -> Product3/1
  Product6/1 -> Add2/1  "Du_p"
  Du/1 -> Data Type Conversion/1
  Product3/1 -> Add1/1  "Du_m"
  Du_sec/1 -> Data Type Conversion1/1
  Add1/1 -> Product6/1  "DutyU"
  [period_reg] -> Multiport Switch/3
  OFF/1 -> Multiport Switch/4
  Du_clamp/1 -> Multiport Switch/1
  Data Type Conversion1/1 -> Add1/2
  Dv_clamp/1 -> Multiport Switch1/1
  Product1/1 -> Add3/1  "Dv_m"
  OFF1/1 -> Multiport Switch1/4
  Data Type Conversion3/1 -> Add3/2
  Add4/1 -> Multiport Switch1/2
  Data Type Conversion2/1 -> Product1/1
  Add3/1 -> Product2/1  "DutyV"
  [period_reg] -> Multiport Switch1/3
  Dv/1 -> Data Type Conversion2/1
  Dv_sec/1 -> Data Type Conversion3/1
  Product2/1 -> Add4/1  "Dv_p"
  [period_reg] -> Shift Arithmetic/1, Product5/2, Product2/2, Product6/2
  Dw_sec/1 -> Data Type Conversion5/1
  M/1 -> Product4/2, Product1/2, Product3/2
  Shift Arithmetic/1 -> Add2/2, Add6/2, Add4/2
  angle/1 -> Dv_clamp/1, Dw_clamp/1, Dw_sec/1, Dw/1, Dv_sec/1, Dv/1, Du_sec/1, Du/1, Du_clamp/1  "angle_ramp"
  [period_reg] -> Multiport Switch2/3
  Data Type Conversion5/1 -> Add5/2
  Add6/1 -> Multiport Switch2/2
  Add5/1 -> Product5/1  "DutyW"
  Dw/1 -> Data Type Conversion4/1
  Dw_clamp/1 -> Multiport Switch2/1
  OFF2/1 -> Multiport Switch2/4
  Product4/1 -> Add5/1  "Dw_m"
  Data Type Conversion4/1 -> Product4/1
  Product5/1 -> Add6/1  "Dw_p"

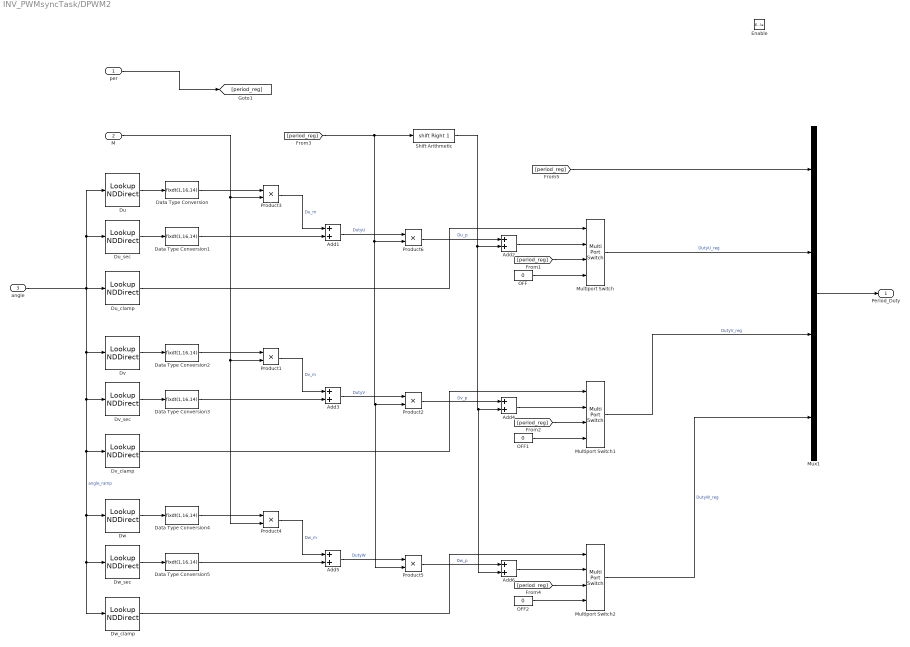
== system INV_PWMsyncTask/DPWM2 ==
  per : Inport
  M : Inport  Port=2
  angle : Inport  Port=3
  Enable : EnablePort
  Add1 : Sum  RndMeth=Simplest  OutDataTypeStr=Inherit: Same as first input
  Add2 : Sum  OutDataTypeStr=uint16  RndMeth=Simplest  SaturateOnIntegerOverflow=on
  Add3 : Sum  RndMeth=Simplest  OutDataTypeStr=Inherit: Same as first input
  Add4 : Sum  OutDataTypeStr=uint16  RndMeth=Simplest  SaturateOnIntegerOverflow=on
  Add5 : Sum  RndMeth=Simplest  OutDataTypeStr=Inherit: Same as first input
  Add6 : Sum  OutDataTypeStr=uint16  RndMeth=Simplest  SaturateOnIntegerOverflow=on
  Data Type Conversion{,1..5} (6 alike) : DataTypeConversion  OutDataTypeStr=fixdt(1,16,14)  ConvertRealWorld=Stored Integer (SI)  RndMeth=Simplest  SaturateOnIntegerOverflow=off
  Du : LookupNDDirect  NumberOfTableDimensions=1  Table=DPWM2Dufi  DiagnosticForOutOfRangeInput=None  RemoveProtectionInput=on  TableDataTypeStr=int16
      settings: LockScale=on
  Du_clamp : LookupNDDirect  NumberOfTableDimensions=1  Table=DPWM2Duclamp  RemoveProtectionInput=on  TableDataTypeStr=uint8
      settings: LockScale=on
  Du_sec : LookupNDDirect  NumberOfTableDimensions=1  Table=DPWM2Dusecfi  RemoveProtectionInput=on  TableDataTypeStr=int16
      settings: LockScale=on
  Dv : LookupNDDirect  NumberOfTableDimensions=1  Table=DPWM2Dvfi  DiagnosticForOutOfRangeInput=None  RemoveProtectionInput=on  TableDataTypeStr=int16
      settings: LockScale=on
  Dv_clamp : LookupNDDirect  NumberOfTableDimensions=1  Table=DPWM2Dvclamp  RemoveProtectionInput=on  TableDataTypeStr=uint8
      settings: LockScale=on
  Dv_sec : LookupNDDirect  NumberOfTableDimensions=1  Table=DPWM2Dvsecfi  RemoveProtectionInput=on  TableDataTypeStr=int16
      settings: LockScale=on
  Dw : LookupNDDirect  NumberOfTableDimensions=1  Table=DPWM2Dwfi  DiagnosticForOutOfRangeInput=None  RemoveProtectionInput=on  TableDataTypeStr=int16
      settings: LockScale=on
  Dw_clamp : LookupNDDirect  NumberOfTableDimensions=1  Table=DPWM2Dwclamp  RemoveProtectionInput=on  TableDataTypeStr=uint8
      settings: LockScale=on
  Dw_sec : LookupNDDirect  NumberOfTableDimensions=1  Table=DPWM2Dwsecfi  RemoveProtectionInput=on  TableDataTypeStr=int16
      settings: LockScale=on
  Multiport Switch : MultiPortSwitch  DataPortOrder=Zero-based contiguous  DiagnosticForDefault=None  zeroidx=on  SaturateOnIntegerOverflow=off  InputSameDT=off
  Multiport Switch1 : MultiPortSwitch  DataPortOrder=Zero-based contiguous  DiagnosticForDefault=None  zeroidx=on  SaturateOnIntegerOverflow=off  InputSameDT=off
  Multiport Switch2 : MultiPortSwitch  DataPortOrder=Zero-based contiguous  DiagnosticForDefault=None  zeroidx=on  SaturateOnIntegerOverflow=off  InputSameDT=off
  Mux1 : Mux
  OFF : Constant  Value=0  OutDataTypeStr=uint16  SampleTime=-1
  OFF1 : Constant  Value=0  OutDataTypeStr=uint16  SampleTime=-1
  OFF2 : Constant  Value=0  OutDataTypeStr=uint16  SampleTime=-1
  Product1 : Product  RndMeth=Simplest  OutDataTypeStr=Inherit: Same as first input  LockScale=on
  Product2 : Product  OutDataTypeStr=int16  RndMeth=Simplest
  Product3 : Product  RndMeth=Simplest  OutDataTypeStr=Inherit: Same as first input  LockScale=on
  Product4 : Product  RndMeth=Simplest  OutDataTypeStr=Inherit: Same as first input  LockScale=on
  Product5 : Product  OutDataTypeStr=int16  RndMeth=Simplest
  Product6 : Product  OutDataTypeStr=int16  RndMeth=Simplest
  Shift Arithmetic : ArithShift  BitShiftNumber=1  BitShiftDirection=Right
  Period_Duty : Outport
  wires:
  [period_reg] -> Mux1/1
  Multiport Switch/1 -> Mux1/2  "DutyU_reg"
  Multiport Switch1/1 -> Mux1/3  "DutyV_reg"
  Multiport Switch2/1 -> Mux1/4  "DutyW_reg"
  Mux1/1 -> Period_Duty/1
  per/1 -> [period_reg]
  Add2/1 -> Multiport Switch/2
  Data Type Conversion/1 -> Product3/1
  Product6/1 -> Add2/1  "Du_p"
  Du/1 -> Data Type Conversion/1
  Product3/1 -> Add1/1  "Du_m"
  Du_sec/1 -> Data Type Conversion1/1
  Add1/1 -> Product6/1  "DutyU"
  [period_reg] -> Multiport Switch/3
  OFF/1 -> Multiport Switch/4
  Du_clamp/1 -> Multiport Switch/1
  Data Type Conversion1/1 -> Add1/2
  Dv_clamp/1 -> Multiport Switch1/1
  Product1/1 -> Add3/1  "Dv_m"
  OFF1/1 -> Multiport Switch1/4
  Data Type Conversion3/1 -> Add3/2
  Add4/1 -> Multiport Switch1/2
  Data Type Conversion2/1 -> Product1/1
  Add3/1 -> Product2/1  "DutyV"
  [period_reg] -> Multiport Switch1/3
  Dv/1 -> Data Type Conversion2/1
  Dv_sec/1 -> Data Type Conversion3/1
  Product2/1 -> Add4/1  "Dv_p"
  [period_reg] -> Shift Arithmetic/1, Product5/2, Product2/2, Product6/2
  Dw_sec/1 -> Data Type Conversion5/1
  M/1 -> Product4/2, Product1/2, Product3/2
  Shift Arithmetic/1 -> Add2/2, Add6/2, Add4/2
  angle/1 -> Dv_clamp/1, Dw_clamp/1, Dw_sec/1, Dw/1, Dv_sec/1, Dv/1, Du_sec/1, Du/1, Du_clamp/1  "angle_ramp"
  [period_reg] -> Multiport Switch2/3
  Data Type Conversion5/1 -> Add5/2
  Add6/1 -> Multiport Switch2/2
  Add5/1 -> Product5/1  "DutyW"
  Dw/1 -> Data Type Conversion4/1
  Dw_clamp/1 -> Multiport Switch2/1
  OFF2/1 -> Multiport Switch2/4
  Product4/1 -> Add5/1  "Dw_m"
  Data Type Conversion4/1 -> Product4/1
  Product5/1 -> Add6/1  "Dw_p"

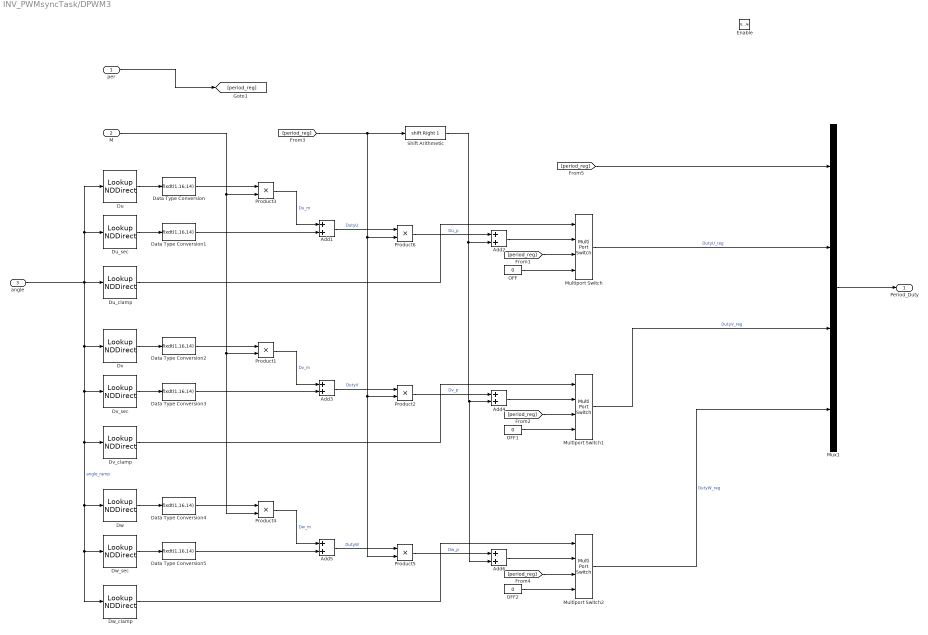
== system INV_PWMsyncTask/DPWM3 ==
  per : Inport
  M : Inport  Port=2
  angle : Inport  Port=3
  Enable : EnablePort
  Add1 : Sum  RndMeth=Simplest  OutDataTypeStr=Inherit: Same as first input
  Add2 : Sum  OutDataTypeStr=uint16  RndMeth=Simplest  SaturateOnIntegerOverflow=on
  Add3 : Sum  RndMeth=Simplest  OutDataTypeStr=Inherit: Same as first input
  Add4 : Sum  OutDataTypeStr=uint16  RndMeth=Simplest  SaturateOnIntegerOverflow=on
  Add5 : Sum  RndMeth=Simplest  OutDataTypeStr=Inherit: Same as first input
  Add6 : Sum  OutDataTypeStr=uint16  RndMeth=Simplest  SaturateOnIntegerOverflow=on
  Data Type Conversion{,1..5} (6 alike) : DataTypeConversion  OutDataTypeStr=fixdt(1,16,14)  ConvertRealWorld=Stored Integer (SI)  RndMeth=Simplest  SaturateOnIntegerOverflow=off
  Du : LookupNDDirect  NumberOfTableDimensions=1  Table=DPWM3Dufi  DiagnosticForOutOfRangeInput=None  RemoveProtectionInput=on  TableDataTypeStr=int16
      settings: LockScale=on
  Du_clamp : LookupNDDirect  NumberOfTableDimensions=1  Table=DPWM3Duclamp  RemoveProtectionInput=on  TableDataTypeStr=uint8
      settings: LockScale=on
  Du_sec : LookupNDDirect  NumberOfTableDimensions=1  Table=DPWM3Dusecfi  RemoveProtectionInput=on  TableDataTypeStr=int16
      settings: LockScale=on
  Dv : LookupNDDirect  NumberOfTableDimensions=1  Table=DPWM3Dvfi  DiagnosticForOutOfRangeInput=None  RemoveProtectionInput=on  TableDataTypeStr=int16
      settings: LockScale=on
  Dv_clamp : LookupNDDirect  NumberOfTableDimensions=1  Table=DPWM3Dvclamp  RemoveProtectionInput=on  TableDataTypeStr=uint8
      settings: LockScale=on
  Dv_sec : LookupNDDirect  NumberOfTableDimensions=1  Table=DPWM3Dvsecfi  RemoveProtectionInput=on  TableDataTypeStr=int16
      settings: LockScale=on
  Dw : LookupNDDirect  NumberOfTableDimensions=1  Table=DPWM3Dwfi  DiagnosticForOutOfRangeInput=None  RemoveProtectionInput=on  TableDataTypeStr=int16
      settings: LockScale=on
  Dw_clamp : LookupNDDirect  NumberOfTableDimensions=1  Table=DPWM3Dwclamp  RemoveProtectionInput=on  TableDataTypeStr=uint8
      settings: LockScale=on
  Dw_sec : LookupNDDirect  NumberOfTableDimensions=1  Table=DPWM3Dwsecfi  RemoveProtectionInput=on  TableDataTypeStr=int16
      settings: LockScale=on
  Multiport Switch : MultiPortSwitch  DataPortOrder=Zero-based contiguous  DiagnosticForDefault=None  zeroidx=on  SaturateOnIntegerOverflow=off  InputSameDT=off
  Multiport Switch1 : MultiPortSwitch  DataPortOrder=Zero-based contiguous  DiagnosticForDefault=None  zeroidx=on  SaturateOnIntegerOverflow=off  InputSameDT=off
  Multiport Switch2 : MultiPortSwitch  DataPortOrder=Zero-based contiguous  DiagnosticForDefault=None  zeroidx=on  SaturateOnIntegerOverflow=off  InputSameDT=off
  Mux1 : Mux
  OFF : Constant  Value=0  OutDataTypeStr=uint16  SampleTime=-1
  OFF1 : Constant  Value=0  OutDataTypeStr=uint16  SampleTime=-1
  OFF2 : Constant  Value=0  OutDataTypeStr=uint16  SampleTime=-1
  Product1 : Product  RndMeth=Simplest  OutDataTypeStr=Inherit: Same as first input  LockScale=on
  Product2 : Product  OutDataTypeStr=int16  RndMeth=Simplest
  Product3 : Product  RndMeth=Simplest  OutDataTypeStr=Inherit: Same as first input  LockScale=on
  Product4 : Product  RndMeth=Simplest  OutDataTypeStr=Inherit: Same as first input  LockScale=on
  Product5 : Product  OutDataTypeStr=int16  RndMeth=Simplest
  Product6 : Product  OutDataTypeStr=int16  RndMeth=Simplest
  Shift Arithmetic : ArithShift  BitShiftNumber=1  BitShiftDirection=Right
  Period_Duty : Outport
  wires:
  [period_reg] -> Mux1/1
  Multiport Switch/1 -> Mux1/2  "DutyU_reg"
  Multiport Switch1/1 -> Mux1/3  "DutyV_reg"
  Multiport Switch2/1 -> Mux1/4  "DutyW_reg"
  Mux1/1 -> Period_Duty/1
  per/1 -> [period_reg]
  Add2/1 -> Multiport Switch/2
  Data Type Conversion/1 -> Product3/1
  Product6/1 -> Add2/1  "Du_p"
  Du/1 -> Data Type Conversion/1
  Product3/1 -> Add1/1  "Du_m"
  Du_sec/1 -> Data Type Conversion1/1
  Add1/1 -> Product6/1  "DutyU"
  [period_reg] -> Multiport Switch/3
  OFF/1 -> Multiport Switch/4
  Du_clamp/1 -> Multiport Switch/1
  Data Type Conversion1/1 -> Add1/2
  Dv_clamp/1 -> Multiport Switch1/1
  Product1/1 -> Add3/1  "Dv_m"
  OFF1/1 -> Multiport Switch1/4
  Data Type Conversion3/1 -> Add3/2
  Add4/1 -> Multiport Switch1/2
  Data Type Conversion2/1 -> Product1/1
  Add3/1 -> Product2/1  "DutyV"
  [period_reg] -> Multiport Switch1/3
  Dv/1 -> Data Type Conversion2/1
  Dv_sec/1 -> Data Type Conversion3/1
  Product2/1 -> Add4/1  "Dv_p"
  [period_reg] -> Shift Arithmetic/1, Product5/2, Product2/2, Product6/2
  Dw_sec/1 -> Data Type Conversion5/1
  M/1 -> Product4/2, Product1/2, Product3/2
  Shift Arithmetic/1 -> Add2/2, Add6/2, Add4/2
  angle/1 -> Dv_clamp/1, Dw_clamp/1, Dw_sec/1, Dw/1, Dv_sec/1, Dv/1, Du_sec/1, Du/1, Du_clamp/1  "angle_ramp"
  [period_reg] -> Multiport Switch2/3
  Data Type Conversion5/1 -> Add5/2
  Add6/1 -> Multiport Switch2/2
  Add5/1 -> Product5/1  "DutyW"
  Dw/1 -> Data Type Conversion4/1
  Dw_clamp/1 -> Multiport Switch2/1
  OFF2/1 -> Multiport Switch2/4
  Product4/1 -> Add5/1  "Dw_m"
  Data Type Conversion4/1 -> Product4/1
  Product5/1 -> Add6/1  "Dw_p"

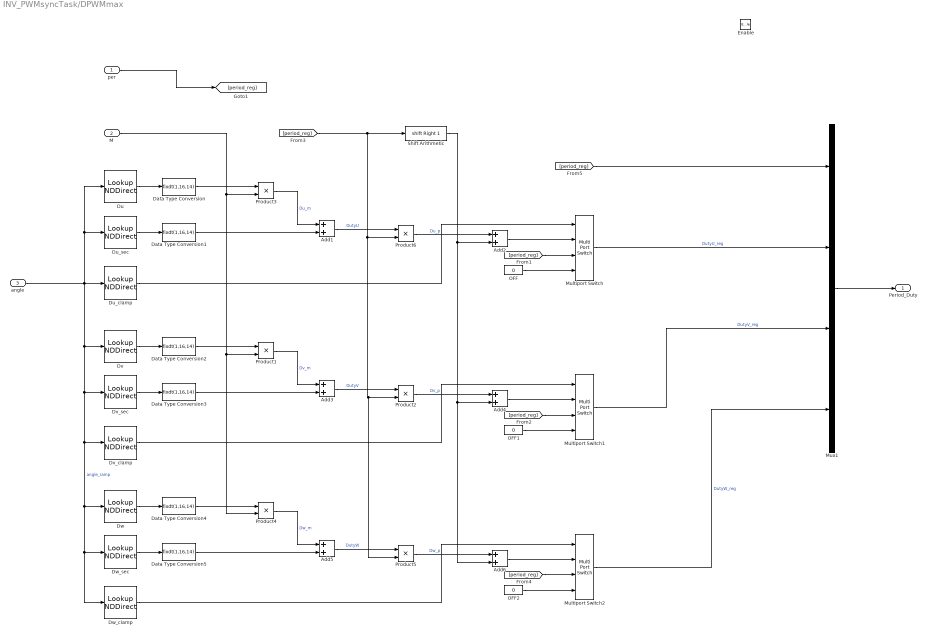
== system INV_PWMsyncTask/DPWMmax ==
  per : Inport
  M : Inport  Port=2
  angle : Inport  Port=3
  Enable : EnablePort
  Add1 : Sum  RndMeth=Simplest  OutDataTypeStr=Inherit: Same as first input
  Add2 : Sum  OutDataTypeStr=uint16  RndMeth=Simplest  SaturateOnIntegerOverflow=on
  Add3 : Sum  RndMeth=Simplest  OutDataTypeStr=Inherit: Same as first input
  Add4 : Sum  OutDataTypeStr=uint16  RndMeth=Simplest  SaturateOnIntegerOverflow=on
  Add5 : Sum  RndMeth=Simplest  OutDataTypeStr=Inherit: Same as first input
  Add6 : Sum  OutDataTypeStr=uint16  RndMeth=Simplest  SaturateOnIntegerOverflow=on
  Data Type Conversion{,1..5} (6 alike) : DataTypeConversion  OutDataTypeStr=fixdt(1,16,14)  ConvertRealWorld=Stored Integer (SI)  RndMeth=Simplest  SaturateOnIntegerOverflow=off
  Du : LookupNDDirect  NumberOfTableDimensions=1  Table=DPWMmaxDufi  DiagnosticForOutOfRangeInput=None  RemoveProtectionInput=on  TableDataTypeStr=int16
      settings: LockScale=on
  Du_clamp : LookupNDDirect  NumberOfTableDimensions=1  Table=DPWMmaxDuclamp  RemoveProtectionInput=on  TableDataTypeStr=uint8
      settings: LockScale=on
  Du_sec : LookupNDDirect  NumberOfTableDimensions=1  Table=DPWMmaxDusecfi  RemoveProtectionInput=on  TableDataTypeStr=int16
      settings: LockScale=on
  Dv : LookupNDDirect  NumberOfTableDimensions=1  Table=DPWMmaxDvfi  DiagnosticForOutOfRangeInput=None  RemoveProtectionInput=on  TableDataTypeStr=int16
      settings: LockScale=on
  Dv_clamp : LookupNDDirect  NumberOfTableDimensions=1  Table=DPWMmaxDvclamp  RemoveProtectionInput=on  TableDataTypeStr=uint8
      settings: LockScale=on
  Dv_sec : LookupNDDirect  NumberOfTableDimensions=1  Table=DPWMmaxDvsecfi  RemoveProtectionInput=on  TableDataTypeStr=int16
      settings: LockScale=on
  Dw : LookupNDDirect  NumberOfTableDimensions=1  Table=DPWMmaxDwfi  DiagnosticForOutOfRangeInput=None  RemoveProtectionInput=on  TableDataTypeStr=int16
      settings: LockScale=on
  Dw_clamp : LookupNDDirect  NumberOfTableDimensions=1  Table=DPWMmaxDwclamp  RemoveProtectionInput=on  TableDataTypeStr=uint8
      settings: LockScale=on
  Dw_sec : LookupNDDirect  NumberOfTableDimensions=1  Table=DPWMmaxDwsecfi  RemoveProtectionInput=on  TableDataTypeStr=int16
      settings: LockScale=on
  Multiport Switch : MultiPortSwitch  DataPortOrder=Zero-based contiguous  DiagnosticForDefault=None  zeroidx=on  SaturateOnIntegerOverflow=off  InputSameDT=off
  Multiport Switch1 : MultiPortSwitch  DataPortOrder=Zero-based contiguous  DiagnosticForDefault=None  zeroidx=on  SaturateOnIntegerOverflow=off  InputSameDT=off
  Multiport Switch2 : MultiPortSwitch  DataPortOrder=Zero-based contiguous  DiagnosticForDefault=None  zeroidx=on  SaturateOnIntegerOverflow=off  InputSameDT=off
  Mux1 : Mux
  OFF : Constant  Value=0  OutDataTypeStr=uint16  SampleTime=-1
  OFF1 : Constant  Value=0  OutDataTypeStr=uint16  SampleTime=-1
  OFF2 : Constant  Value=0  OutDataTypeStr=uint16  SampleTime=-1
  Product1 : Product  RndMeth=Simplest  OutDataTypeStr=Inherit: Same as first input  LockScale=on
  Product2 : Product  OutDataTypeStr=int16  RndMeth=Simplest
  Product3 : Product  RndMeth=Simplest  OutDataTypeStr=Inherit: Same as first input  LockScale=on
  Product4 : Product  RndMeth=Simplest  OutDataTypeStr=Inherit: Same as first input  LockScale=on
  Product5 : Product  OutDataTypeStr=int16  RndMeth=Simplest
  Product6 : Product  OutDataTypeStr=int16  RndMeth=Simplest
  Shift Arithmetic : ArithShift  BitShiftNumber=1  BitShiftDirection=Right
  Period_Duty : Outport
  wires:
  Multiport Switch2/1 -> Mux1/4  "DutyW_reg"
  Multiport Switch1/1 -> Mux1/3  "DutyV_reg"
  Multiport Switch/1 -> Mux1/2  "DutyU_reg"
  [period_reg] -> Mux1/1
  Mux1/1 -> Period_Duty/1
  per/1 -> [period_reg]
  Add2/1 -> Multiport Switch/2
  Data Type Conversion/1 -> Product3/1
  Product6/1 -> Add2/1  "Du_p"
  Du/1 -> Data Type Conversion/1
  Product3/1 -> Add1/1  "Du_m"
  Du_sec/1 -> Data Type Conversion1/1
  Add1/1 -> Product6/1  "DutyU"
  [period_reg] -> Multiport Switch/3
  OFF/1 -> Multiport Switch/4
  Du_clamp/1 -> Multiport Switch/1
  Data Type Conversion1/1 -> Add1/2
  Dv_clamp/1 -> Multiport Switch1/1
  Product1/1 -> Add3/1  "Dv_m"
  OFF1/1 -> Multiport Switch1/4
  Data Type Conversion3/1 -> Add3/2
  Add4/1 -> Multiport Switch1/2
  Data Type Conversion2/1 -> Product1/1
  Add3/1 -> Product2/1  "DutyV"
  [period_reg] -> Multiport Switch1/3
  Dv/1 -> Data Type Conversion2/1
  Dv_sec/1 -> Data Type Conversion3/1
  Product2/1 -> Add4/1  "Dv_p"
  [period_reg] -> Shift Arithmetic/1, Product5/2, Product2/2, Product6/2
  Dw_sec/1 -> Data Type Conversion5/1
  M/1 -> Product4/2, Product1/2, Product3/2
  Shift Arithmetic/1 -> Add2/2, Add6/2, Add4/2
  angle/1 -> Dv_clamp/1, Dw_clamp/1, Dw_sec/1, Dw/1, Dv_sec/1, Dv/1, Du_sec/1, Du/1, Du_clamp/1  "angle_ramp"
  [period_reg] -> Multiport Switch2/3
  Data Type Conversion5/1 -> Add5/2
  Add6/1 -> Multiport Switch2/2
  Add5/1 -> Product5/1  "DutyW"
  Dw/1 -> Data Type Conversion4/1
  Dw_clamp/1 -> Multiport Switch2/1
  OFF2/1 -> Multiport Switch2/4
  Product4/1 -> Add5/1  "Dw_m"
  Data Type Conversion4/1 -> Product4/1
  Product5/1 -> Add6/1  "Dw_p"
